simulink model "lolz_cascading"  (R2017a)
settings: Solver=VariableStepAuto  StartTime=0.0  StopTime=5  RelTol=1e-3
undefined symbols (not defined in the file): A, B, Discrete, K, kalman_C, kalman_D, kalman_R, Time
libraries: ctrlSharedLib x1
settings Model: Creator=keith  LastModifiedBy=keith

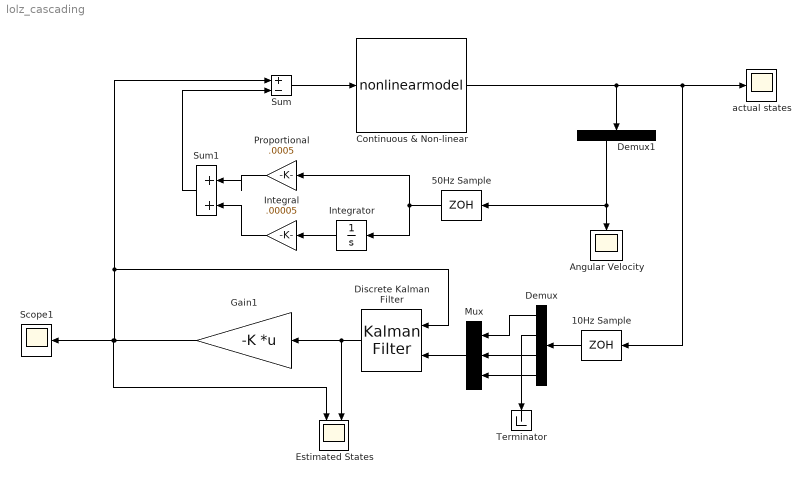
== system lolz_cascading ==
  10Hz Sample : ZeroOrderHold  SampleTime=.1
  50Hz Sample : ZeroOrderHold  SampleTime=.02
  Angular Velocity : Scope
  Continuous & Non-linear : S-Function  InitFcn=try, set_param(gcb,'FunctionName','nonlinearmodel'), end  FunctionName=nonlinearmodel  SFunctionModules=nonlinearmodel_wrapper  SFunctionDeploymentMode=off  EnableBusSupport=off  mask(S-Function Builder){}
      mask help: Simulink:masks:SFunctionBuilder_MD
      mask init:
      | val = [[.9  0.75 0.75 1 1 .9 .9 1]',[1 1 0.75 0.75 .9 .9 1 .9]'];try , sys = get_param(gcb,'SfunBuilderFcnName');if isempty(sys), sys = get_param(gcb,'FunctionName'); end,catch, sys = get_param(gcb,'FunctionName'); end
      settings: CopyFcn=set_param(gcbh,'LinkStatus','none')  PreSaveFcn=try, set_param(gcb,'FunctionName','nonlinearmodel'), end  OpenFcn=sfunctionwizard(gcbh)
      mask Display: plot(val(:,1),val(:,2)),disp(sys), port_label('input',1,'u0'), port_label('output',1,'y0')
  Demux : Demux
  Demux1 : Demux
  Discrete Kalman Filter : ctrlSharedLib/Kalman Filter  TimeDomain=Discrete-Time  UseCurrentEstimator=on  ModelSource=Individual A, B, C, D matrices  ModelSourceVariable=ss(0.95,1,1,0,1)  A=A  B=B  C=kalman_C  D=kalman_D  NumberOfStates=1  NumberOfInputs=1  NumberOfOutputs=1  InitialEstimateSource=Dialog  X0=[0;0;0;0]  P0=10  UseK=off  UseGH=off  NumberOfProcessNoiseInputs=1  G=1  TimeInvariantG=on  H=0  TimeInvariantH=on  Q=0.05  TimeInvariantQ=on  R=kalman_R  TimeInvariantR=on  N=0  TimeInvariantN=on  AddInputPort=on  AddEnablePort=off  OutputEstimatedY=off  OutputP=off  Ts=-1
  Estimated States : Scope  NumInputPorts=2
  Gain1 : Gain  Gain=-K  Multiplication=Matrix(K*u)
  Integral : Gain  Gain=.00005
  Integrator : Integrator
  Mux : Mux  Inputs=3
  Proportional : Gain  Gain=.0005
  Scope1 : Scope
  Sum : Sum  Inputs=+-
  Sum1 : Sum  Inputs=|++
  Terminator : Terminator
  actual states : Scope
  wires:
  Continuous & Non-linear/1 -> Demux1/1, actual states/1, 10Hz Sample/1
  Gain1/1 -> Scope1/1, Estimated States/1, Sum/1, Discrete Kalman Filter/1
  Discrete Kalman Filter/1 -> Estimated States/2, Gain1/1
  10Hz Sample/1 -> Demux/1
  Mux/1 -> Discrete Kalman Filter/2
  Demux/1 -> Mux/1
  Demux/3 -> Mux/2
  Demux/4 -> Mux/3
  Demux/2 -> Terminator/1
  Demux1/2 -> 50Hz Sample/1, Angular Velocity/1
  Sum/1 -> Continuous & Non-linear/1
  50Hz Sample/1 -> Proportional/1, Integrator/1
  Integrator/1 -> Integral/1
  Proportional/1 -> Sum1/1
  Integral/1 -> Sum1/2
  Sum1/1 -> Sum/2
